simulink model "err_rpy"  (R2018b)
settings: Solver=FixedStepAuto  StartTime=t_start  StopTime=t_end  FixedStep=Ts  RelTol=1e-3
values from neighbouring files (symbols this model uses):
  ARSP_time = data.ARSP(:,2)/1000    [err_rpym.m]
  ATT_PitchSensor = data.ATT(:,6)/100/180*pi    [err_rpym.m]
  ATT_RollSensor = data.ATT(:,4)/100/180*pi    [err_rpym.m]
  ATT_time = data.ATT(:,2)/1000    [err_rpym.m]
  ATT_YawSensor = data.ATT(:,8)/100/180*pi    [err_rpym.m]
  GPS_time = data1.data(:,1)    [err_rpym.m]
  GPS_VX = data1.data(:,5)    [err_rpym.m]
  GPS_VY = data1.data(:,6)    [err_rpym.m]
  GPS_VZ = data1.data(:,7)    [err_rpym.m]
  IMU_accel = data.IMU(:,6:8)    [err_rpym.m]
  IMU_time = data.IMU(:,2)/1000    [err_rpym.m]
  Ts = 0.1    [err_rpym.m]
undefined symbols (not defined in the file or in its folder): ARSP_speed_x, ARSP_speed_y, GPS_cog
settings Model: Creator=a4327  LastModifiedBy=a4327

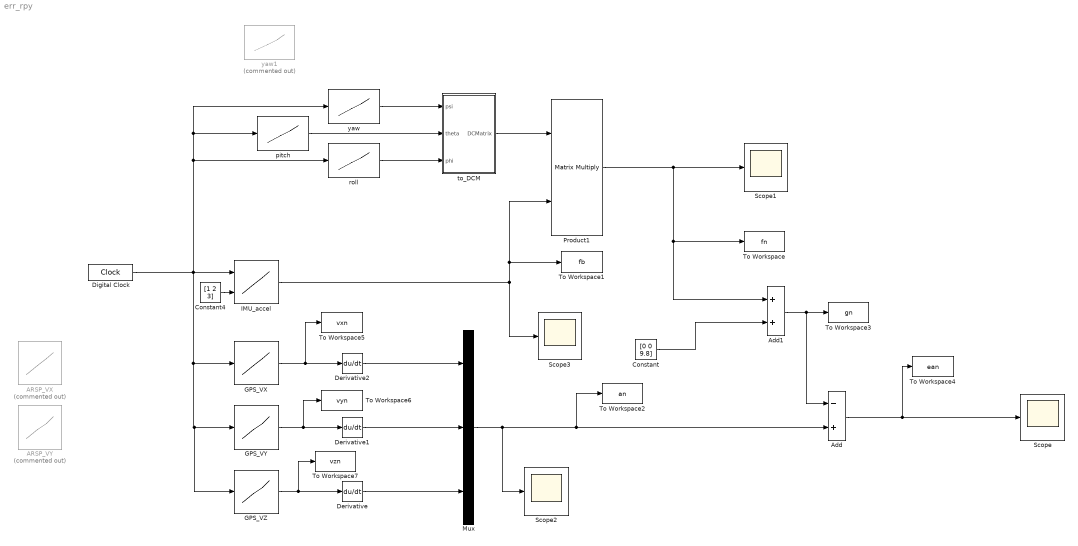
== system err_rpy ==
  ARSP_VX : Lookup_n-D  Commented=on  NumberOfTableDimensions=1  BreakpointsForDimension1=ARSP_time  Table=ARSP_speed_x  InternalRulePriority=Speed  RndMeth=Simplest  InputSameDT=on
  ARSP_VY : Lookup_n-D  Commented=on  NumberOfTableDimensions=1  BreakpointsForDimension1=ARSP_time  Table=ARSP_speed_y  InternalRulePriority=Speed  RndMeth=Simplest  InputSameDT=on
  Add : Sum  Inputs=-+
  Add1 : Sum
  Constant : Constant  Value=[0 0 9.8]
  Constant4 : Constant  Value=[1 2 3]
  Derivative : Derivative
  Derivative1 : Derivative
  Derivative2 : Derivative
  Digital Clock : DigitalClock  SampleTime=Ts
  GPS_VX : Lookup_n-D  NumberOfTableDimensions=1  BreakpointsForDimension1=GPS_time  Table=GPS_VX  InternalRulePriority=Speed  RndMeth=Simplest  InputSameDT=on
  GPS_VY : Lookup_n-D  NumberOfTableDimensions=1  BreakpointsForDimension1=GPS_time  Table=GPS_VY  InternalRulePriority=Speed  RndMeth=Simplest  InputSameDT=on
  GPS_VZ : Lookup_n-D  NumberOfTableDimensions=1  BreakpointsForDimension1=GPS_time  Table=GPS_VZ  InternalRulePriority=Speed  RndMeth=Simplest  InputSameDT=on
  IMU_accel : Lookup_n-D  BreakpointsForDimension1=IMU_time  BreakpointsForDimension2=[1,2,3]  Table=IMU_accel  InternalRulePriority=Speed  RndMeth=Simplest  InputSameDT=on
  Mux : Mux  Inputs=3
  Product1 : Product  Multiplication=Matrix(*)
  Scope{,1..3} (4 alike) : Scope
  To Workspace : ToWorkspace  VariableName=fn  SaveFormat=Structure With Time  SampleTime=-1
  To Workspace1 : ToWorkspace  VariableName=fb  SaveFormat=Structure With Time  SampleTime=-1
  To Workspace2 : ToWorkspace  VariableName=an  SaveFormat=Structure With Time  SampleTime=-1
  To Workspace3 : ToWorkspace  VariableName=gn  SaveFormat=Structure With Time  SampleTime=-1
  To Workspace4 : ToWorkspace  VariableName=ean  SaveFormat=Structure With Time  SampleTime=-1
  To Workspace5 : ToWorkspace  VariableName=vxn  SaveFormat=Structure With Time  SampleTime=-1
  To Workspace6 : ToWorkspace  VariableName=vyn  SaveFormat=Structure With Time  SampleTime=-1
  To Workspace7 : ToWorkspace  VariableName=vzn  SaveFormat=Structure With Time  SampleTime=-1
  pitch : Lookup_n-D  NumberOfTableDimensions=1  BreakpointsForDimension1=ATT_time  Table=ATT_PitchSensor  InternalRulePriority=Speed  RndMeth=Simplest  InputSameDT=on
  roll : Lookup_n-D  NumberOfTableDimensions=1  BreakpointsForDimension1=ATT_time  Table=ATT_RollSensor  InternalRulePriority=Speed  RndMeth=Simplest  InputSameDT=on
  to_DCM : Subsystem
  yaw : Lookup_n-D  NumberOfTableDimensions=1  BreakpointsForDimension1=ATT_time  Table=ATT_YawSensor  InternalRulePriority=Speed  RndMeth=Simplest  InputSameDT=on
  yaw1 : Lookup_n-D  Commented=on  NumberOfTableDimensions=1  BreakpointsForDimension1=GPS_time  Table=GPS_cog  InternalRulePriority=Speed  RndMeth=Simplest  InputSameDT=on
  wires:
  to_DCM/1(DCMatrix) -> Product1/1
  GPS_VZ/1 -> To Workspace7/1, Derivative/1
  GPS_VY/1 -> To Workspace6/1, Derivative1/1
  GPS_VX/1 -> To Workspace5/1, Derivative2/1
  Digital Clock/1 -> yaw/1, pitch/1, roll/1, GPS_VZ/1, GPS_VY/1, GPS_VX/1, IMU_accel/1
  Constant4/1 -> IMU_accel/2
  IMU_accel/1 -> Scope3/1, Product1/2, To Workspace1/1
  yaw/1 -> to_DCM/1(psi)
  pitch/1 -> to_DCM/2(theta)
  roll/1 -> to_DCM/3(phi)
  Derivative2/1 -> Mux/1
  Derivative1/1 -> Mux/2
  Derivative/1 -> Mux/3
  Mux/1 -> To Workspace2/1, Add/2, Scope2/1
  Add/1 -> To Workspace4/1, Scope/1
  Product1/1 -> Add1/1, To Workspace/1, Scope1/1
  Constant/1 -> Add1/2
  Add1/1 -> Add/1, To Workspace3/1

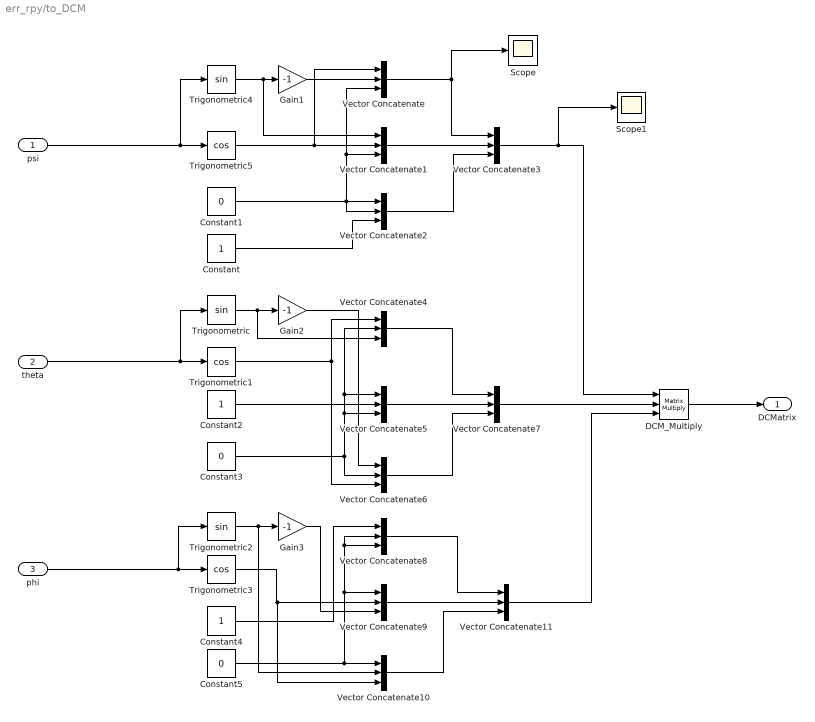
== system err_rpy/to_DCM ==
  psi : Inport
  theta : Inport  Port=2
  phi : Inport  Port=3
  Constant : Constant
  Constant1 : Constant  Value=0
  Constant2 : Constant
  Constant3 : Constant  Value=0
  Constant4 : Constant
  Constant5 : Constant  Value=0
  DCM_Multiply : Product  Inputs=3  Multiplication=Matrix(*)
  Gain1 : Gain  Gain=-1
  Gain2 : Gain  Gain=-1
  Gain3 : Gain  Gain=-1
  Scope : Scope
  Scope1 : Scope
  Trigonometric : Trigonometry
  Trigonometric1 : Trigonometry  Operator=cos
  Trigonometric2 : Trigonometry
  Trigonometric3 : Trigonometry  Operator=cos
  Trigonometric4 : Trigonometry
  Trigonometric5 : Trigonometry  Operator=cos
  Vector Concatenate{,1..2,4..6,8..10} (9 alike) : Concatenate  NumInputs=3  Mode=Multidimensional array  ConcatenateDimension=2
  Vector Concatenate11 : Concatenate  NumInputs=3  Mode=Multidimensional array
  Vector Concatenate3 : Concatenate  NumInputs=3  Mode=Multidimensional array
  Vector Concatenate7 : Concatenate  NumInputs=3  Mode=Multidimensional array
  DCMatrix : Outport
  wires:
  Vector Concatenate1/1 -> Vector Concatenate3/2
  Vector Concatenate2/1 -> Vector Concatenate3/3
  Constant2/1 -> Vector Concatenate5/2
  Vector Concatenate10/1 -> Vector Concatenate11/3
  Gain2/1 -> Vector Concatenate6/1
  Gain3/1 -> Vector Concatenate9/3
  Vector Concatenate5/1 -> Vector Concatenate7/2
  Constant4/1 -> Vector Concatenate8/1
  Constant5/1 -> Vector Concatenate10/1, Vector Concatenate9/1, Vector Concatenate8/2, Vector Concatenate8/3
  Vector Concatenate8/1 -> Vector Concatenate11/1
  Vector Concatenate9/1 -> Vector Concatenate11/2
  Vector Concatenate6/1 -> Vector Concatenate7/3
  Vector Concatenate4/1 -> Vector Concatenate7/1
  Constant3/1 -> Vector Concatenate6/2, Vector Concatenate4/2, Vector Concatenate5/1, Vector Concatenate5/3
  Constant/1 -> Vector Concatenate2/3
  theta/1 -> Trigonometric1/1, Trigonometric/1
  phi/1 -> Trigonometric2/1, Trigonometric3/1
  Trigonometric1/1 -> Vector Concatenate6/3, Vector Concatenate4/1
  Trigonometric3/1 -> Vector Concatenate10/3, Vector Concatenate9/2
  psi/1 -> Trigonometric5/1, Trigonometric4/1
  Trigonometric2/1 -> Vector Concatenate10/2, Gain3/1
  Constant1/1 -> Vector Concatenate1/3, Vector Concatenate/3, Vector Concatenate2/2, Vector Concatenate2/1
  DCM_Multiply/1 -> DCMatrix/1
  Trigonometric4/1 -> Vector Concatenate1/1, Gain1/1
  Trigonometric5/1 -> Vector Concatenate1/2, Vector Concatenate/1
  Trigonometric/1 -> Vector Concatenate4/3, Gain2/1
  Gain1/1 -> Vector Concatenate/2
  Vector Concatenate3/1 -> Scope1/1, DCM_Multiply/1
  Vector Concatenate7/1 -> DCM_Multiply/2
  Vector Concatenate11/1 -> DCM_Multiply/3
  Vector Concatenate/1 -> Scope/1, Vector Concatenate3/1
